simulink model "excneuron"  (Simulink 7.6)
settings: Solver=ode45  StartTime=0.0  StopTime=10.0  RelTol=1e-3
values from neighbouring files (symbols this model uses):
  h = -0.5    [excneuroninit.m]
  maxcon = 10    [excneuroninit.m]
  neurodist = 1    [excneuroninit.m]
  sigslope = 3    [excneuroninit.m]
  tau_u = 0.05    [excneuroninit.m]
libraries: simulink x1
settings Model: Creator=root  LastModifiedBy=root

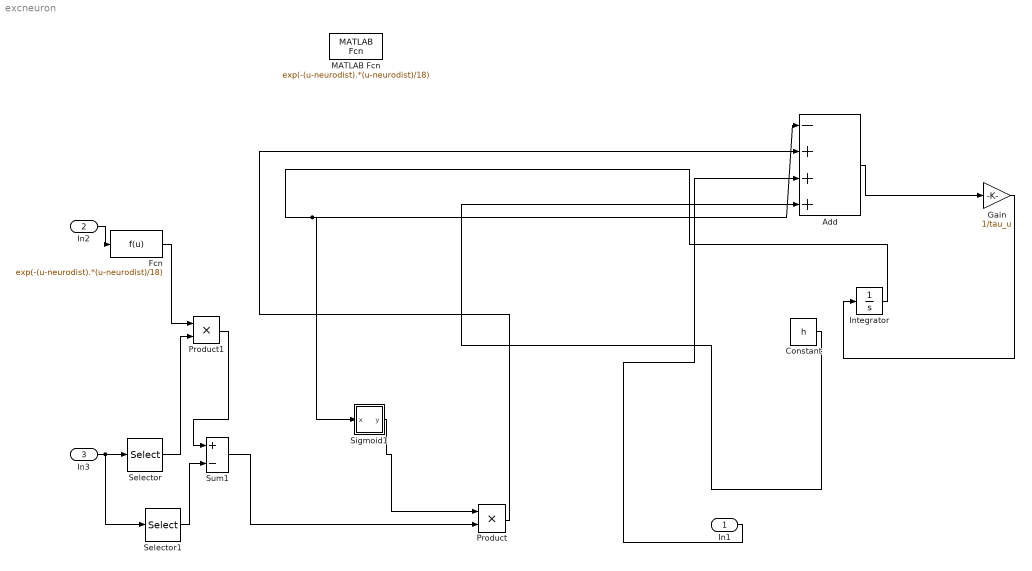
== system excneuron ==
  In1 : Inport
  In2 : Inport  Port=2
  In3 : Inport  Port=3
  Add : Sum  Inputs=-+++
  Constant : Constant  Value=h
  Fcn : Fcn  Expr=exp(-(u-neurodist).*(u-neurodist)/18)
  Gain : Gain  Gain=1/tau_u
  Integrator : Integrator
  MATLAB Fcn : MATLABFcn  MATLABFcn=exp(-(u-neurodist).*(u-neurodist)/18)  OutputDimensions=maxcon
  Product : Product  RndMeth=Zero
  Product1 : Product  RndMeth=Zero
  Selector : Selector  InputPortWidth=maxcon+1  IndexOptions=Starting index (dialog)  Indices=2  OutputSizes=maxcon
  Selector1 : Selector  InputPortWidth=maxcon+1  IndexOptions=Starting index (dialog)  Indices=1  OutputSizes=1
  Sigmoid1 : Subsystem  TreatAsAtomicUnit=on  mask{slope=sigslope, offset=0}
      mask help: Created by Han, Cheol
      mask Display: plot([10 15 20 25 30 35 40 45 50], [0 0.01 0.1 0.2 0.5 0.8 0.9 0.99 1])
  Sum1 : Sum  Inputs=+-  SaturateOnIntegerOverflow=on
  wires:
  Add/1 -> Gain/1
  Gain/1 -> Integrator/1
  Integrator/1 -> Add/1, Sigmoid1/1(x)
  Sigmoid1/1(y) -> Product/1
  Product/1 -> Add/2
  In1/1 -> Add/3
  Constant/1 -> Add/4
  In3/1 -> Selector/1, Selector1/1
  Selector/1 -> Product1/2
  Product1/1 -> Sum1/1
  Selector1/1 -> Sum1/2
  Sum1/1 -> Product/2
  In2/1 -> Fcn/1
  Fcn/1 -> Product1/1

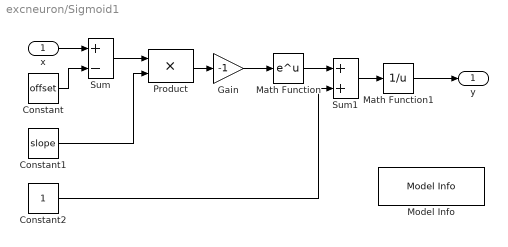
== system excneuron/Sigmoid1 ==
  x : Inport
  Constant : Constant  Value=offset
  Constant1 : Constant  Value=slope
  Constant2 : Constant
  Gain : Gain  Gain=-1  SaturateOnIntegerOverflow=on  OutDataTypeStr=Inherit: Same as input  ParamDataTypeStr=Inherit: Same as input
  Math Function : Math  SaturateOnIntegerOverflow=on
  Math Function1 : Math  Operator=reciprocal  SaturateOnIntegerOverflow=on
  Model Info : simulink/Model-Wide Utilities/Model Info  SystemSampleTime=-1  InitialBlockCM=None  BlockCM=None  Frame=on  DisplayStringWithTags=|  HorizontalTextAlignment=Center  LeftAlignmentValue=0.5  SourceBlockDiagram=excneuron  TagMaxNumber=20
      | Model Info
      | %<Creator> Han, Cheol
  Product : Product  SaturateOnIntegerOverflow=on  OutDataTypeStr=Inherit: Same as first input
  Sum : Sum  Inputs=+-  SaturateOnIntegerOverflow=on
  Sum1 : Sum  SaturateOnIntegerOverflow=on
  y : Outport  InitialOutput=0
  wires:
  x/1 -> Sum/1
  Constant/1 -> Sum/2
  Sum/1 -> Product/1
  Constant1/1 -> Product/2
  Product/1 -> Gain/1
  Gain/1 -> Math Function/1
  Math Function/1 -> Sum1/1
  Constant2/1 -> Sum1/2
  Sum1/1 -> Math Function1/1
  Math Function1/1 -> y/1
